simulink model "proj2_3_ship1"  (Simulink 7.4)
settings: Solver=ode3  StartTime=0.0  StopTime=30.0  RelTol=1e-3
libraries: vipgeotforms x2, viptextngfix x1, vipconversions x1, vipsrcs x1, vipsnks x1
settings Model: Creator=piepmeie  LastModifiedBy=m134506

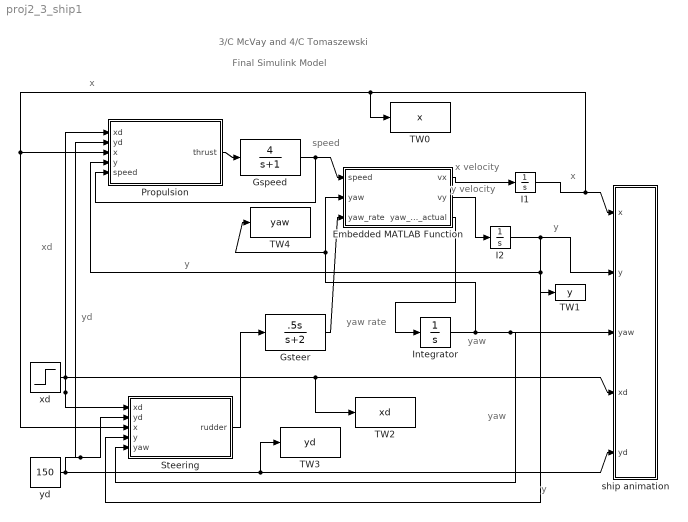
== system proj2_3_ship1 ==
  note: x
  note: y
  note: x velocity
  note: y velocity
  note: speed
  note: yaw
  note: yaw rate
  note: y
  note: x
  note: xd
  note: yd
  note: yaw
  note: y
  note: 3/C McVay and 4/C Tomaszewski
  note: Final Simulink Model
  Embedded MATLAB Function : Stateflow chart
  Gspeed : TransferFcn  Numerator=[4]  Denominator=[1 1]
  Gsteer : TransferFcn  Numerator=[.5 0]  Denominator=[1 2]
  I1 : Integrator
  I2 : Integrator
  Integrator : Integrator  InitialCondition=pi/4
  Propulsion : Stateflow chart
  Steering : Stateflow chart
  TW0 : ToWorkspace  VariableName=x  SampleTime=-1  SaveFormat=Array
  TW1 : ToWorkspace  VariableName=y  SampleTime=-1  SaveFormat=Array
  TW2 : ToWorkspace  VariableName=xd  SampleTime=-1  SaveFormat=Array
  TW3 : ToWorkspace  VariableName=yd  SampleTime=-1  SaveFormat=Array
  TW4 : ToWorkspace  VariableName=yaw  SampleTime=-1  SaveFormat=Array
  ship animation : Subsystem
  xd : Step  Time=13  After=-100  SampleTime=0
  yd : Constant  Value=150  OutDataType=fixdt(1, 16)  OutScaling=2^0
  wires:
  Propulsion/1(thrust) -> Gspeed/1
  Steering/1(rudder) -> Gsteer/1
  Gsteer/1 -> Embedded MATLAB Function/3(yaw_rate)
  Integrator/1 -> ship animation/3(yaw), Steering/5(yaw), Embedded MATLAB Function/2(yaw), TW4/1
  Gspeed/1 -> Embedded MATLAB Function/1(speed), Propulsion/5(speed)
  Embedded MATLAB Function/1(vx) -> I1/1
  I1/1 -> ship animation/1(x), Steering/3(x), Propulsion/3(x), TW0/1
  Embedded MATLAB Function/2(vy) -> I2/1
  I2/1 -> ship animation/2(y), Steering/4(y), Propulsion/4(y), TW1/1
  xd/1 -> Steering/1(xd), ship animation/4(xd), TW2/1, Propulsion/1(xd)
  yd/1 -> Steering/2(yd), Propulsion/2(yd), ship animation/5(yd), TW3/1
  Embedded MATLAB Function/3(yaw_rate_actual) -> Integrator/1

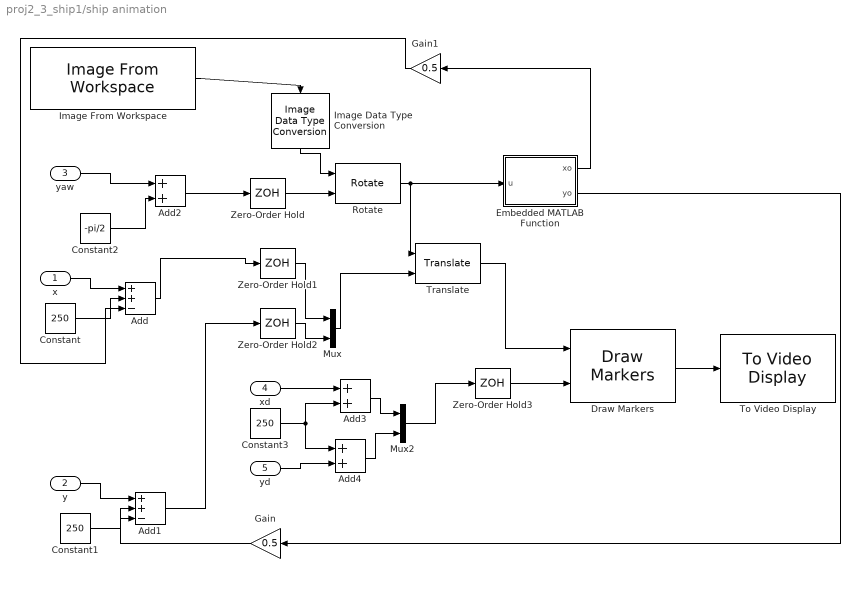
== system proj2_3_ship1/ship animation ==
  x : Inport  OutDataType=sfix(16)  OutScaling=2^0
  y : Inport  Port=2  OutDataType=sfix(16)  OutScaling=2^0
  yaw : Inport  Port=3  OutDataType=sfix(16)  OutScaling=2^0
  xd : Inport  Port=4  OutDataType=sfix(16)  OutScaling=2^0
  yd : Inport  Port=5  OutDataType=sfix(16)  OutScaling=2^0
  Add : Sum  Inputs=++-  OutDataType=sfix(16)  OutScaling=2^-10
  Add1 : Sum  Inputs=++-  OutDataType=sfix(16)  OutScaling=2^-10
  Add2 : Sum  OutDataType=sfix(16)  OutScaling=2^-10
  Add3 : Sum  OutDataType=sfix(16)  OutScaling=2^-10
  Add4 : Sum  OutDataType=sfix(16)  OutScaling=2^-10
  Constant : Constant  Value=250  OutDataType=sfix(16)  OutScaling=2^0
  Constant1 : Constant  Value=250  OutDataType=sfix(16)  OutScaling=2^0
  Constant2 : Constant  Value=-pi/2  OutDataType=sfix(16)  OutScaling=2^0
  Constant3 : Constant  Value=250  OutDataType=sfix(16)  OutScaling=2^0
  Draw Markers : viptextngfix/Draw Markers  DialogController=vipDDGCreate  DialogControllerArgs=DataTag0  shape=X-mark  size=6  fill=off  fillClrSource=Specify via dialog  display=White  intensity=155  color=[200 120 50]  opacity=1  viewport=Entire image  antialiasing=off  inType=Obsolete  imagePorts=One multidimensional signal  prodOutputMode=Binary point scaling  prodOutputWordLength=32  prodOutputFracLength=14  memoryMode=Specify word length  memoryWordLength=16  memoryFracLength=15  roundingMode=Floor  overflowMode=off
  Embedded MATLAB Function : Stateflow chart  TreatAsAtomicUnit=on
  Gain : Gain  Gain=0.5  ParameterDataType=sfix(16)  ParameterScaling=2^0  OutDataType=sfix(16)  OutScaling=2^0
  Gain1 : Gain  Gain=0.5  ParameterDataType=sfix(16)  ParameterScaling=2^0  OutDataType=sfix(16)  OutScaling=2^0
  Image Data Type Conversion : vipconversions/Image Data Type Conversion  outDT=double  isSigned=on  wordLen=16  numFracBits=0
  Image From Workspace : vipsrcs/Image From Workspace  Tag=vipblks_nd  SystemSampleTime=-1  ImageValue=ship  Ts=inf  imagePorts=One multidimensional signal  ImageDataType=Inherit from 'Value'  Signed=on  WordLength=16  sdImageDataType=sfix(16)  FractionLengthMode=User-defined  FractionLength=15  OutPortLabels=R|G|B
  Mux : Mux  Inputs=2
  Mux2 : Mux  Inputs=2
  Rotate : vipgeotforms/Rotate  DialogController=vipDDGCreate  DialogControllerArgs=DataTag1  outSizeR=Expanded to fit rotated input image  src_angle=Input port  unit_angle=Degrees  angle=pi/6  maxAngle=pi  dispImage=Center  method=Table lookup  fillVal=0  interpMethod=Bilinear  prodOutputMode=Binary point scaling  prodOutputWordLength=32  prodOutputFracLength=10  roundingMode=Nearest  overflowMode=on
  To Video Display : vipsnks/To Video Display  DialogControllerArgs=DataTag2  inputType=Obsolete  imagePorts=One multidimensional signal  OutputDevice=On-screen video monitor  fullScreen=off  videoWindowX=1008  videoWindowY=21  saveWindowSize=off  videoWindowWidth=594  videoWindowHeight=595  dataOrg=Column-major  openAtMdlStart=on  isWindowOpen=on
  Translate : vipgeotforms/Translate  DialogController=vipDDGCreate  DialogControllerArgs=DataTag3  outSizeT=Full  src_trans=Input port  translation="[1.5  2.3]"  maxOffset=[500 500]  fillVal=0  interpMethod=Bilinear  prodOutputMode=Binary point scaling  prodOutputWordLength=32  prodOutputFracLength=10  roundingMode=Nearest  overflowMode=on
  Zero-Order Hold{,1..3} (4 alike) : ZeroOrderHold  SampleTime=1/30
  wires:
  Image From Workspace/1 -> Image Data Type Conversion/1
  Image Data Type Conversion/1 -> Rotate/1
  Zero-Order Hold/1 -> Rotate/2
  Zero-Order Hold2/1 -> Mux/2
  Zero-Order Hold1/1 -> Mux/1
  Mux/1 -> Translate/2
  Constant/1 -> Add/2
  Constant1/1 -> Add1/2
  Add/1 -> Zero-Order Hold1/1
  Add1/1 -> Zero-Order Hold2/1
  Constant2/1 -> Add2/2
  Add2/1 -> Zero-Order Hold/1
  Translate/1 -> Draw Markers/1
  Draw Markers/1 -> To Video Display/1
  Rotate/1 -> Embedded MATLAB Function/1(u), Translate/1
  Embedded MATLAB Function/2(yo) -> Gain/1
  Gain/1 -> Add1/3
  Embedded MATLAB Function/1(xo) -> Gain1/1
  Gain1/1 -> Add/3
  x/1 -> Add/1
  y/1 -> Add1/1
  yaw/1 -> Add2/1
  Zero-Order Hold3/1 -> Draw Markers/2
  xd/1 -> Add3/1
  yd/1 -> Add4/2
  Add4/1 -> Mux2/2
  Add3/1 -> Mux2/1
  Constant3/1 -> Add3/2, Add4/1
  Mux2/1 -> Zero-Order Hold3/1

== matlab function ship animation/Embedded MATLAB Function ==
  data: u input double; xo output double; yo output double
function [xo, yo] = fcn(u)
% This block supports the Embedded MATLAB subset.
% See the help menu for details. 

K = size(u);
xo = K(1);
yo = K(2);

== matlab function Embedded MATLAB Function ==
  data: speed input double; vx output double; yaw input double; vy output double; yaw_rate input double; yaw_rate_actual output double
function [vx,vy,yaw_rate_actual] = real_dynamics(speed,yaw,yaw_rate)

vx=speed*cos(yaw);
vy=speed*sin(yaw);
yaw_rate_actual=speed*0.03*yaw_rate;

== matlab function Steering ==
  data: xd input double; yd input double; x input double; y input double; yaw input double; rudder output double
function rudder  = steering(xd,yd,x,y,yaw)

Ksteer=75;
yawd=atan2((yd-y),(xd-x)); %desired yaw value
yaw_err=yawd-yaw;          %error in yaw
while(abs(yaw_err)>pi)     %while trying to go long way
    yaw_err=-sign(yaw_err)*2*pi+yaw_err; %add/subtract 2*pi
end
rudder=Ksteer*(yaw_err);  %base rudder angle shortest turn

== matlab function Propulsion ==
  data: xd input double; yd input double; x input double; y input double; thrust output double; speed input double
function thrust = propulsion(xd,yd,x,y,speed)

Kd=8;
Kthrust=4;
if((abs(xd-x)<.1)&&(abs(yd-y)<.1))
    thrust=0;
%elseif((abs(xd-x)<2)&&(abs(yd-y)<2))
    %thrust=0.8*(sqrt((xd-x)^2+(yd-y)^2))-Kd*speed;
else
    thrust=Kthrust*(sqrt((xd-x)^2+(yd-y)^2))-Kd*speed;
end
